simulink model "TuneCurrentControl"  (R2020b)
settings: Solver=VariableStepAuto  StartTime=0.0  StopTime=10.0  RelTol=1e-3
undefined symbols (not defined in the file): DiscIntNeverNeededParam, plant_Jmotor, plant_Kb, plant_Kt, plant_L, plant_R
libraries: simulink x2, slctrlblks x1
settings Model: DataDictionary=Dictionary.sldd  EnableAccessToBaseWorkspace=off  Creator=alons  LastModifiedBy=alons

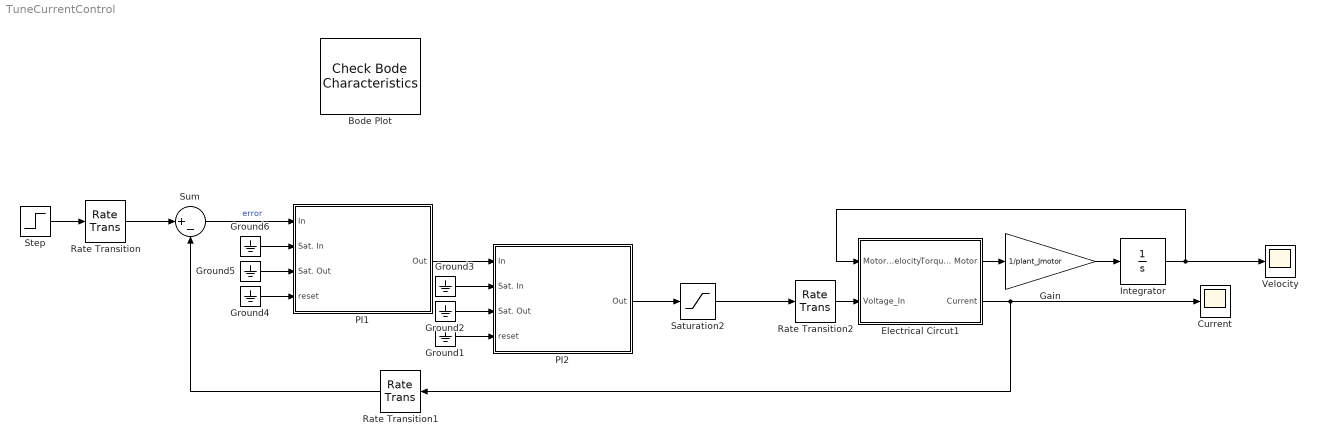
== system TuneCurrentControl ==
  Bode Plot : slctrlblks/Model Verification/Check Bode  Characteristics  InstantiateOnLoad=on  SaveOperatingPoints=off  LinearizationIOs={'/Sum', 1, 'in', 'off', '';'/Electrical Circut', 2, 'out', 'off', ''}  LinearizeAt=SnapshotTimes  SnapshotTimes=[0]  TriggerType=rising  SampleTime=auto  RateConversionMethod=zoh  PreWarpFreq=10  UseExactDelayModel=off  UseFullBlockNameLabels=off  UseBusSignalLabels=off  enabled=on  stopWhenAssertionFail=off  export=off  ViewDlgPos=[100 200 510 390]  OpenViewOnLoad=off  LaunchViewOnOpen=off  FrequencyUnits=rad/s  MagnitudeUnits=dB  PhaseUnits=deg  TimeUnits=seconds  EnableUpperBound=off  UpperBoundFrequencies=[]  UpperBoundMagnitudes=[]  EnableLowerBound=off  LowerBoundFrequencies=[]  LowerBoundMagnitudes=[]
  Current : Scope
  Electrical Circut1 : Subsystem  mask{K_T=plant_Kt, K_b=plant_Kb, R=plant_R, L=plant_L}
      mask prompts: K_T "K_T [Nm/A]"; K_b "K_b[Vpeak/(rad/s)]"; R "R [Ohm]"; L "L [H]"
      mask init:
      | set_param(gcbh,'backgroundcolor','brown' );
      mask Display:
      | x=0.05+[ 0.4781
      |     0.2730
      |     0.4435
      |     0.2984
      |     0.4412
      |     0.3514
      |     0.5910
      |     0.4435
      |     0.5818
      |     0.4182
      |     0.4781];
      | 
      | y=[ 0.9111
      |     0.5875
      |     0.5816
      |     0.3192
      |     0.3338
      |     0.0423
      |     0.4009
      |     0.4009
      |     0.6516
      |     0.6516
      |     0.9082];
      | 
      | patch(x,y,[0.8,0.7,0.1])
      | plot(x,y)
  Gain : Gain  Gain=1/plant_Jmotor
  Ground{1..6} (6 alike) : Ground
  Integrator : Integrator
  PI1 : Subsystem  mask{a=30, K=1, awup_en=off, EN=on}
      mask prompts: a "PI Zero [Hz] (a)"; K "PI Gain (K)"; awup_en "Anti-WindUp"; EN "Enable"
      mask help:
      | PI Controller of the form:
      |
      | K*(s + a*2*pi)
      |     ---------------
      |            s
      mask init:
      | if EN %strcmp(enable_block,'on')~=(sw_on=='1')
      | 	set_param(gcbh,'backgroundcolor','orange');
      | else
      | 	set_param(gcbh,'backgroundcolor','gray');
      | end
      | 
      | s = get_param(gcb,'maskvalues');
      | num_s =  ['[1 ',num2str(s{1}), '*2*pi]'];
      | den_s  = ['[1 0]'];
      | 
      | gain = ['[' num2str(s{2}) ']'];
      | zero = ['[-' num2str(s{1}), '*2*pi]'];
      | pole = '[0]';
      settings: AttributesFormatString="PI %<a>Hz  Gain = %<K>"
      mask Display: droots(zero,pole,gain)
  PI2 : Subsystem  mask{a=30, K=1, awup_en=off, EN=on}
      mask prompts: a "PI Zero [Hz] (a)"; K "PI Gain (K)"; awup_en "Anti-WindUp"; EN "Enable"
      mask help:
      | PI Controller of the form:
      |
      | K*(s + a*2*pi)
      |     ---------------
      |            s
      mask init: same as TuneCurrentControl/PI1
      settings: AttributesFormatString="PI %<a>Hz  Gain = %<K>"
      mask Display: droots(zero,pole,gain)
  Rate Transition : RateTransition  OutPortSampleTime=ts_control
  Rate Transition1 : RateTransition  OutPortSampleTime=ts_control
  Rate Transition2 : RateTransition  OutPortSampleTime=0
  Saturation2 : Saturate  UpperLimit=10  LowerLimit=-10
      settings: AttributesFormatString=max = %<UpperLimit> [V]\nmin = %<LowerLimit> [V]
  Step : Step  SampleTime=0
  Sum : Sum  Inputs=|+-
  Velocity : Scope
  wires:
  PI2/1(Out) -> Saturation2/1
  Integrator/1 -> Electrical Circut1/1(Motor Velocity), Velocity/1
  Step/1 -> Rate Transition/1
  Ground1/1 -> PI2/4(reset)
  Ground2/1 -> PI2/3(Sat. Out)
  Ground3/1 -> PI2/2(Sat. In)
  Ground4/1 -> PI1/4(reset)
  Ground6/1 -> PI1/2(Sat. In)
  Ground5/1 -> PI1/3(Sat. Out)
  PI1/1(Out) -> PI2/1(In)
  Sum/1 -> PI1/1(In)  "error"
  Saturation2/1 -> Rate Transition2/1
  Gain/1 -> Integrator/1
  Electrical Circut1/1(Torque on Motor) -> Gain/1
  Electrical Circut1/2(Current) -> Current/1, Rate Transition1/1
  Rate Transition/1 -> Sum/1
  Rate Transition1/1 -> Sum/2
  Rate Transition2/1 -> Electrical Circut1/2(Voltage_In)

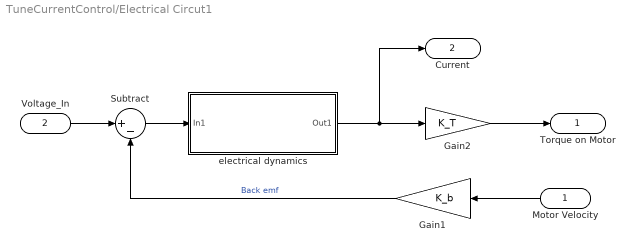
== system TuneCurrentControl/Electrical Circut1 ==
  Motor Velocity : Inport
  Voltage_In : Inport  Port=2
  Gain1 : Gain  Gain=K_b
  Gain2 : Gain  Gain=K_T
  Subtract : Sum  Inputs=|+-
  electrical dynamics : Subsystem
      mask Display: disp('1\n----------\nLs+R')
  Torque on Motor : Outport
  Current : Outport  Port=2
  wires:
  Gain2/1 -> Torque on Motor/1
  Voltage_In/1 -> Subtract/1
  Gain1/1 -> Subtract/2  "Back emf"
  Subtract/1 -> electrical dynamics/1(In1)
  electrical dynamics/1(Out1) -> Current/1, Gain2/1
  Motor Velocity/1 -> Gain1/1

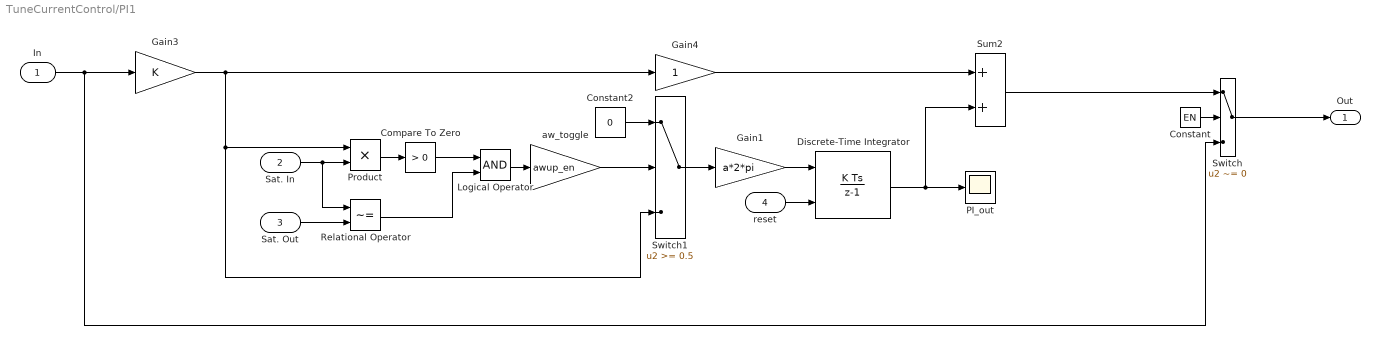
== system TuneCurrentControl/PI1 ==
  In : Inport
  Sat. In : Inport  Port=2
  Sat. Out : Inport  Port=3
  reset : Inport  Port=4
  Compare To Zero : simulink/Logic and Bit Operations/Compare To Zero  relop=>  OutDataTypeStr=boolean
  Constant : Constant  Value=EN
  Constant2 : Constant  Value=0  OutDataTypeStr=Inherit: Inherit via back propagation
  Discrete-Time Integrator : DiscreteIntegrator  ExternalReset=rising  SampleTime=-1  UpperSaturationLimit=4/100  LowerSaturationLimit=-4/100  ICPrevOutput=DiscIntNeverNeededParam  ICPrevScaledInput=DiscIntNeverNeededParam
  Gain1 : Gain  Gain=a*2*pi  SaturateOnIntegerOverflow=on  OutDataTypeStr=Inherit: Same as input  ParamDataTypeStr=Inherit: Same as input
  Gain3 : Gain  Gain=K  SaturateOnIntegerOverflow=on  OutDataTypeStr=Inherit: Same as input  ParamDataTypeStr=Inherit: Same as input
  Gain4 : Gain  SaturateOnIntegerOverflow=on  OutDataTypeStr=Inherit: Same as input  ParamDataTypeStr=Inherit: Same as input
  Logical Operator : Logic  AllPortsSameDT=off  OutDataTypeStr=boolean
  PI_out : Scope
  Product : Product
  Relational Operator : RelationalOperator  Operator=~=  OutDataTypeStr=boolean  RndMeth=Nearest
  Sum2 : Sum  InputSameDT=on  SaturateOnIntegerOverflow=on  OutDataTypeStr=Inherit: Same as first input
  Switch : Switch  Criteria=u2 ~= 0  SaturateOnIntegerOverflow=on
  Switch1 : Switch  Threshold=0.5
  aw_toggle : Gain  Gain=awup_en  SaturateOnIntegerOverflow=on  OutDataTypeStr=Inherit: Same as input  ParamDataTypeStr=Inherit: Same as input
      settings: AttributesFormatString=%<Gain>
  Out : Outport
  wires:
  Gain1/1 -> Discrete-Time Integrator/1
  Gain4/1 -> Sum2/1
  Discrete-Time Integrator/1 -> Sum2/2, PI_out/1
  In/1 -> Switch/3, Gain3/1
  Constant/1 -> Switch/2
  Sum2/1 -> Switch/1
  Switch/1 -> Out/1
  Product/1 -> Compare To Zero/1
  Compare To Zero/1 -> Logical Operator/1
  Relational Operator/1 -> Logical Operator/2
  Logical Operator/1 -> aw_toggle/1
  Gain3/1 -> Switch1/3, Product/1, Gain4/1
  Sat. In/1 -> Product/2, Relational Operator/1
  Sat. Out/1 -> Relational Operator/2
  aw_toggle/1 -> Switch1/2
  Switch1/1 -> Gain1/1
  Constant2/1 -> Switch1/1
  reset/1 -> Discrete-Time Integrator/2

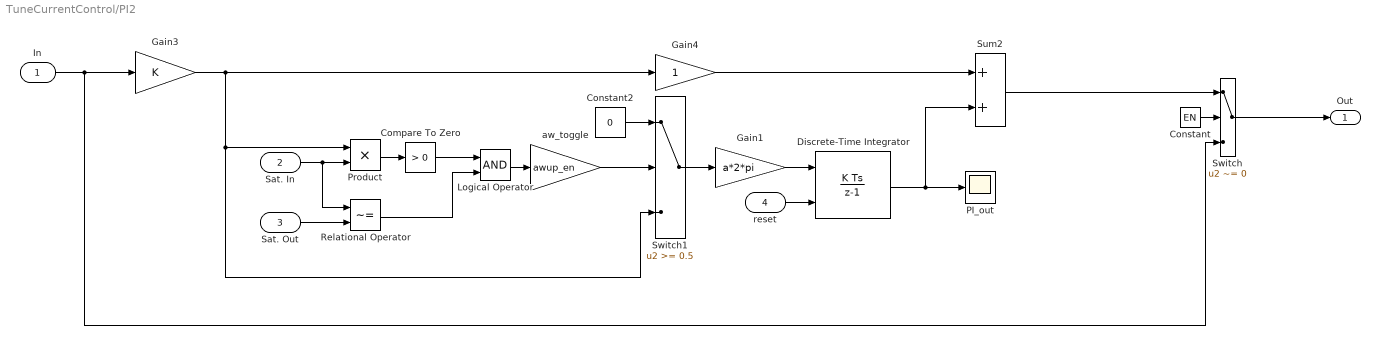
== system TuneCurrentControl/PI2 ==
  In : Inport
  Sat. In : Inport  Port=2
  Sat. Out : Inport  Port=3
  reset : Inport  Port=4
  Compare To Zero : simulink/Logic and Bit Operations/Compare To Zero  relop=>  OutDataTypeStr=boolean
  Constant : Constant  Value=EN
  Constant2 : Constant  Value=0  OutDataTypeStr=Inherit: Inherit via back propagation
  Discrete-Time Integrator : DiscreteIntegrator  ExternalReset=rising  SampleTime=-1  UpperSaturationLimit=4/100  LowerSaturationLimit=-4/100  ICPrevOutput=DiscIntNeverNeededParam  ICPrevScaledInput=DiscIntNeverNeededParam
  Gain1 : Gain  Gain=a*2*pi  SaturateOnIntegerOverflow=on  OutDataTypeStr=Inherit: Same as input  ParamDataTypeStr=Inherit: Same as input
  Gain3 : Gain  Gain=K  SaturateOnIntegerOverflow=on  OutDataTypeStr=Inherit: Same as input  ParamDataTypeStr=Inherit: Same as input
  Gain4 : Gain  SaturateOnIntegerOverflow=on  OutDataTypeStr=Inherit: Same as input  ParamDataTypeStr=Inherit: Same as input
  Logical Operator : Logic  AllPortsSameDT=off  OutDataTypeStr=boolean
  PI_out : Scope
  Product : Product
  Relational Operator : RelationalOperator  Operator=~=  OutDataTypeStr=boolean  RndMeth=Nearest
  Sum2 : Sum  InputSameDT=on  SaturateOnIntegerOverflow=on  OutDataTypeStr=Inherit: Same as first input
  Switch : Switch  Criteria=u2 ~= 0  SaturateOnIntegerOverflow=on
  Switch1 : Switch  Threshold=0.5
  aw_toggle : Gain  Gain=awup_en  SaturateOnIntegerOverflow=on  OutDataTypeStr=Inherit: Same as input  ParamDataTypeStr=Inherit: Same as input
      settings: AttributesFormatString=%<Gain>
  Out : Outport
  wires:
  Gain1/1 -> Discrete-Time Integrator/1
  Gain4/1 -> Sum2/1
  Discrete-Time Integrator/1 -> Sum2/2, PI_out/1
  In/1 -> Switch/3, Gain3/1
  Constant/1 -> Switch/2
  Sum2/1 -> Switch/1
  Switch/1 -> Out/1
  Product/1 -> Compare To Zero/1
  Compare To Zero/1 -> Logical Operator/1
  Relational Operator/1 -> Logical Operator/2
  Logical Operator/1 -> aw_toggle/1
  Gain3/1 -> Switch1/3, Product/1, Gain4/1
  Sat. In/1 -> Product/2, Relational Operator/1
  Sat. Out/1 -> Relational Operator/2
  aw_toggle/1 -> Switch1/2
  Switch1/1 -> Gain1/1
  Constant2/1 -> Switch1/1
  reset/1 -> Discrete-Time Integrator/2

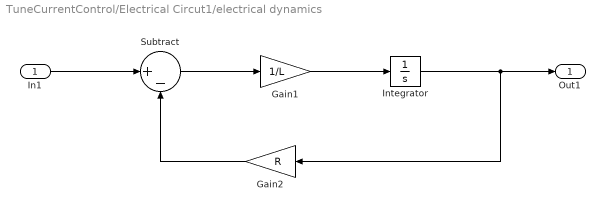
== system TuneCurrentControl/Electrical Circut1/electrical dynamics ==
  In1 : Inport
  Gain1 : Gain  Gain=1/L
  Gain2 : Gain  Gain=R
  Integrator : Integrator
  Subtract : Sum  Inputs=|+-
  Out1 : Outport
  wires:
  In1/1 -> Subtract/1
  Gain1/1 -> Integrator/1
  Subtract/1 -> Gain1/1
  Gain2/1 -> Subtract/2
  Integrator/1 -> Gain2/1, Out1/1
